simulink model "HyQ2Max_Leg_2Dof_ForAc1CylMot"  (Simulink 7.0)
settings: Solver=ode15s  StartTime=0.0  StopTime=10.0  MaxStep=1e-2  RelTol=1e-3
values from neighbouring files (symbols this model uses):
  L_LegInertiab_CAD = [ ... (first row only)    [HyQ2Max_CAD_For_SimMechanics_LF_RF.m]
  L_LegMb = 1.406    [HyQ2Max_CAD_For_SimMechanics_LF_RF.m]
  U_LegInertia_CAD = [0.010196 0.002320 0.000141 ... (first row only)    [HyQ2Max_CAD_For_SimMechanics_LF_RF.m]
  U_LegM = 4.95    [HyQ2Max_CAD_For_SimMechanics_LF_RF.m]
undefined symbols (not defined in the file or in its folder): sigbuilder_block
libraries: mblibv1 x24, fl_lib x15, nesl_utility x6, simulink x2
settings Model: Creator=Gustavo  LastModifiedBy=Gustavo
settings SolverCC: SolverResetMethod=Robust
settings DebuggingCC: SaveWithParameterizedLinksMsg=none  SignalResolutionControl=TryResolveAllWithWarning  MultiTaskDSMMsg=warning  MultiTaskCondExecSysMsg=none
settings RTWCC: IncludeERTFirstTime=on
settings GRTTargetCC: TargetFcnLib=ansi_tfl_tmw.mat
settings SimMechanicsCC: VisOnUpdateDiagram=on  VisDuringSimulation=on

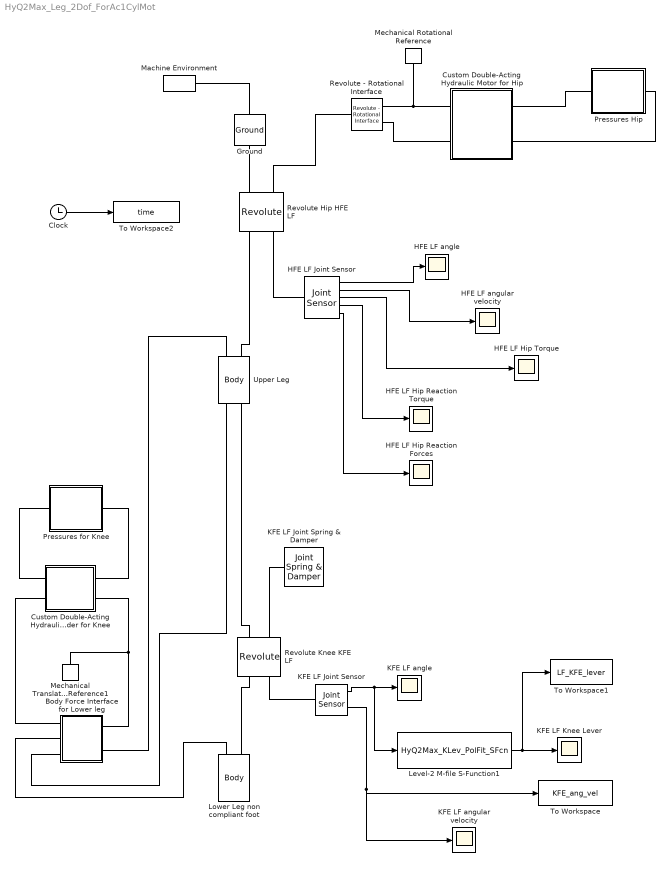
== system HyQ2Max_Leg_2Dof_ForAc1CylMot ==
  Body Force Interface for Lower leg : Subsystem
  Clock : Clock
      settings: Decimation=10
  Custom Double-Acting Hydraulic Cylinder for Knee : Subsystem  Orientation=left  mask(Hydraulic Double-Acting Cylinder, Custom Model){area_A=3.14e-004, area_B=2.00e-004, stroke=0.06834, init_pos=-1.4570e-4, stiffness=1e7, damping=1e5}
      mask prompts: area_A "Area A (m^2)"; area_B "Area B (m^2)"; stroke "Stroke (m)"; init_pos "Initial position (m)"; stiffness "Contact stiffness (N/m)"; damping "Contact damping (N*s/m)"
      mask help: The model is built entirely of Foundation Library blocks and accounts for hard stops and fluid consumption due to piston motion.
      mask Display:
      | plot([127.790967235342;156.136468285695;156.136468285695;127.790967235342;127.790967235342], [113.618216710165;113.618216710165;56.927214609459;56.927214609459;113.618216710165])
      | plot([227.000220911577;227.000220911577;56.927214609459;56.927214609459;227.000220911577;227.000220911577], [99.4454661849886;113.618216710165;113.618216710165;56.927214609459;56.927214609459;71.0999651346356])
      | plot([156.136468285695;297.86397353746;297.86397353746;156.136468285695;156.136468285695], [99.4454661849886;99.4454661849886;71.0999651346356;71.0999651346356;99.4454661849886])
      | plot([56.927214609459;28.581713559106;56.927214609459], [113.618216710165;85.2727156598121;56.927214609459])
      | plot([28.581713559106;0.236212508752942], [85.2727156598121;85.2727156598121])
      | plot([297.86397353746;326.209474587813], [85.2727156598121;85.2727156598121])
      | plot([0.236212508752942;71.0999651346356;71.0999651346356], [28.581713559106;28.581713559106;56.927214609459])
      | plot([212.827470386401;212.827470386401;323.374924482778], [56.927214609459;28.581713559106;28.581713559106])
      | patch([0;326.445687096566;326.445687096566;0;0;0.472425017505884;0.472425017505884;325.97326207906;325.97326207906;0.472425017505884;0], [113.854429218918;113.854429218918;0;0;113.854429218918;113.382004201412;0.472425017505884;0.472425017505884;113.382004201412;113.382004201412;113.854429218918], [1;1;1])
      | ;
  Custom Double-Acting Hydraulic Motor for Hip : Subsystem  Orientation=left  mask(Hydraulic Double-Acting Cylinder, Custom Model){Displacement=1.432e-5, stroke=270/180*pi, init_pos=135/180*pi, stiffness=1e7, damping=1e5, Damping_Coef=1.5}
      mask prompts: Displacement "Displacement (m^3/rad)"; stroke "Stroke (rad)"; init_pos "Initial position (rad)"; stiffness "Contact stiffness (Nm/rad)"; damping "Contact damping (Nm*s/rad)"; Damping_Coef "Damping Coef (Nm*s/rad)"
      mask help: The model is built entirely of Foundation Library blocks and accounts for hard stops and fluid consumption due to piston motion.
      mask Display:
      | plot([73.6992110911092;78.3372264117062;83.4855098283815;89.0944805574945;95.1101211447486;101.474497682805;108.12631774648;115.001520672305;122.033894497737;129.15571361855;136.298391023429;143.39313882438;150.371630721695;157.166660023573;163.712786883295;169.946968520725;175.809166358744;181.242924227569;186.195912068529;190.620429901137;194.473867199977;197.719113257359;200.324914579718;202.266175875843;203.524201738252;204.086876690183;203.948781864259;203.111247189144;201.582338581603;199.376780267312;196.51581297852;193.02698939418;188.943908792596;184.305893471999;179.157610055324;173.548639326211;167.532998738957;161.1686222009;154.516802137226;147.6415992114;140.609225385968;133.487406265155;126.344728860276;119.249981059326;112.27148916201;105.476459860132;98.9303330004107;92.6961513629807;86.8339535249614;81.4001956561362;76.4472078151762;72.0226899825683;70.8644989508936], [212.831540230622;218.265298099447;223.218285940407;227.642803773015;231.496241071855;234.741487129237;237.347288451596;239.288549747721;240.54657561013;241.109250562061;240.971155736137;240.133621061022;238.604712453481;236.39915413919;233.538186850398;230.049363266058;225.966282664474;221.328267343877;216.179983927202;210.571013198089;204.555372610835;198.190996072778;191.539176009104;184.663973083278;177.631599257846;170.509780137033;163.367102732154;156.272354931204;149.293863033888;142.49883373201;135.952706872289;129.718525234859;123.856327396839;118.422569528014;113.469581687054;109.045063854446;105.191626555606;101.946380498224;99.3405791758655;97.3993178797401;96.1412920173311;95.5786170654003;95.7167118913243;96.5542465664391;98.0831551739803;100.288713488271;103.149680777063;106.638504361403;110.721584962987;115.359600283584;120.50788370026;126.116854429373;127.792411177503])
      | plot([0;133.223854936659;133.223854936659], [255.34572196193;255.34572196193;241.172971436754])
      | plot([73.6983027309179;133.223854936659;70.8637526258826], [212.827470386401;170.309218810871;127.790967235342])
      | patch([110.547454096377;153.065705671906;133.223854936659;110.547454096377], [238.338421331719;238.338421331719;209.992920281366;238.338421331719], [0;0;0])
      | plot([110.547454096377;153.065705671906;133.223854936659;110.547454096377], [238.338421331719;238.338421331719;209.992920281366;238.338421331719])
      | patch([110.547454096377;153.065705671906;133.223854936659;110.547454096377], [99.4454661849887;99.4454661849887;127.790967235342;99.4454661849887], [0;0;0])
      | plot([110.547454096377;153.065705671906;133.223854936659;110.547454096377], [99.4454661849887;99.4454661849887;127.790967235342;99.4454661849887])
      | plot([204.087607562542;240.936758928001;240.936758928001;204.087607562542;204.087607562542], [178.812869125977;178.812869125977;161.805568495765;161.805568495765;178.812869125977])
      | plot([5.66910021007061;133.223854936659;133.223854936659], [85.2727156598121;85.2727156598121;96.6109160799534])
      | plot([240.936758928001;283.455010503531], [170.309218810871;170.309218810871])
      | patch([2.59833759628236;286.525773117319;286.525773117319;2.59833759628236;2.59833759628236;3.07076261378825;3.07076261378825;286.053348099813;286.053348099813;3.07076261378825;2.59833759628236], [340.618437621743;340.618437621743;0;5.6843418860808e-14;340.618437621743;340.146012604237;0.472425017505941;0.472425017505884;340.146012604237;340.146012604237;340.618437621743], [1;1;1])
      | ;color('red');
  Ground : mblibv1/Bodies/Ground  Orientation=down  DialogController=MECH.DynMechDlgSource  SystemSampleTime=-1  LeftPortType=env  RightPortType=workingframe  PhysicalDomain=Mechanical  DialogClass=GroundBlock  CoordPosition=[0 0 0]  CoordPositionUnits=m  StateVectorMgrId=-1  MachineId=[0 0]  ShowEnvPort=on
  HFE LF Joint Sensor : mblibv1/Sensors &  Actuators/Joint Sensor  DialogController=MECH.DynMechDlgSource  SystemSampleTime=-1  PhysicalDomain=Mechanical  PortType=blob  Muxed=off  Pose=off  Angle=on  AngleUnits=rad  ArcVelocity=on  ArcVelocityUnits=rad/s  ArcAcceleration=off  ArcAccelerationUnits=rad/s^2  CoordPosition=on  CoordPositionUnits=m  Velocity=off  VelocityUnits=m/s  Acceleration=off  AccelerationUnits=m/s^2  Quaternion=on  QuaternionDT=off  QuaternionDDT=off  QuaternionUnits=off  OutputVector=[ 1 ]  ActiveIO=on  Width=9  DialogClass=MechanicalSensorBlock  Primitive=R1  Force=off  ForceUnits=N  Torque=on  TorqueUnits=N*m  ReferenceFrame=Absolute (INERTIAL)  ReactionSensedSide=Base  ReactionReferenceFrame=Absolute (World)  ReactionForce=on  ReactionForceUnits=N  ReactionMoment=on  ReactionMomentUnits=N*m
  HFE LF angular velocity : Scope
      settings: YMin=-2.5  YMax=0.25  SaveName=ScopeData10
  HFE LF Hip Reaction Forces : Scope
      settings: TimeRange=10  YMin=-40  YMax=40  SaveName=ScopeData6
  HFE LF Hip Reaction Torque : Scope
      settings: TimeRange=10  YMin=-0.4  YMax=0.3  SaveName=ScopeData7
  HFE LF Hip Torque : Scope
      settings: TimeRange=10  YMin=-7.5  YMax=7.5  SaveName=ScopeData4
  HFE LF angle : Scope
      settings: YMin=-2.5  YMax=0.25
  KFE LF Joint Sensor : mblibv1/Sensors &  Actuators/Joint Sensor  DialogController=MECH.DynMechDlgSource  SystemSampleTime=-1  PhysicalDomain=Mechanical  PortType=blob  Muxed=off  Pose=off  Angle=on  AngleUnits=rad  ArcVelocity=on  ArcVelocityUnits=rad/s  ArcAcceleration=off  ArcAccelerationUnits=rad/s^2  CoordPosition=on  CoordPositionUnits=m  Velocity=off  VelocityUnits=m/s  Acceleration=off  AccelerationUnits=m/s^2  Quaternion=on  QuaternionDT=off  QuaternionDDT=off  QuaternionUnits=off  OutputVector=[ 1 ]  ActiveIO=on  Width=2  DialogClass=MechanicalSensorBlock  Primitive=R1  Force=off  ForceUnits=N  Torque=off  TorqueUnits=N*m  ReferenceFrame=Absolute (INERTIAL)  ReactionSensedSide=Base  ReactionReferenceFrame=Absolute (World)  ReactionForce=off  ReactionForceUnits=N  ReactionMoment=off  ReactionMomentUnits=N*m
  KFE LF Joint Spring & Damper : mblibv1/Force  Elements/Joint Spring & Damper  DialogController=MECH.DynMechDlgSource  SystemSampleTime=-1  DialogClass=JointSpringDamper  JFEParameters=P1$false$0$0$0$m$m/s$N$deg$deg/s$N*m#P2$false$0$0$0$m$m/s$N$deg$deg/s$N*m#P3$false$0$0$0$m$m/s$N$deg$deg/s$N*m#R1$true$0$0.5$0$m$m/s$N$rad$rad/s$N*m#R2$false$0$0$0$m$m/s$N$deg$deg/s$N*m#R3$false$0$0$0$m$m/s$N$deg$deg/s$N*m#S$false$0$0$0$m$m/s$N$deg$deg/s$N*m
  KFE LF Knee Lever : Scope
      settings: TimeRange=10  YMin=0.005  YMax=0.04  SaveName=ScopeData9
  KFE LF angle : Scope
      settings: YMin=-3.5  YMax=3.5  SaveName=ScopeData8
  KFE LF angular velocity : Scope
      settings: YMin=-3.5  YMax=3.5
  Level-2 M-file S-Function1 : M-S-Function  FunctionName=HyQ2Max_KLev_PolFit_SFcn
  Lower Leg non compliant foot : mblibv1/Bodies/Body  Orientation=down  DialogController=MECH.DynMechDlgSource  PhysicalDomain=mechanical  SubClassName=Unknown  LeftPortType=workingframe  RightPortType=workingframe  LConnTagsString=CS3|CS1  RConnTagsString=CS2  DialogClass=MechanicalBodyBlock  Mass=L_LegMb  MassUnits=kg  InertiaUnits=kg*m^2  Inertia=L_LegInertiab_CAD  Shape=Cylinder  ShapeDims=[1 1]  ShapeUnits=m  ShapeUse=false  Density=1  DensityUnits=kg/m^3  DensityUse=false  CG=Left$CG$L_LegCogb_CAD$CS1$CS1$m$[-90 180 0]$Euler Z-X-Z$deg$World$false  WorkingFrames="Left$CS3$[0.0262 0.0216 0]$CS1$CS1$m$[-90 180 0]$Euler Z-X-Z$deg$World$true#Left$CS1$[0 0  0]$Adjoining$Adjoining$m$[-90 180 0]$Euler Z-X-Z$deg$World$true#Right$CS2$[0.38009 0 0]$CS1$CS1$m$[-90 180 0]$Euler Z-X-Z$deg$World$true"  CGPos=L_LegCogb_CAD  CGRot=[-90 180 0]  CS0Pos=[]  CS0Rot=[]  CS1Pos="[0 0  0]"  CS1Rot=[-90 180 0]  CS2Pos=[0.38009 0 0]  CS2Rot=[-90 180 0]  CS3Pos=[0.0262 0.0216 0]  CS3Rot=[-90 180 0]  CS4Pos=[]  CS4Rot=[]  CS5Pos=[]  CS5Rot=[]  CS6Pos=[]  CS6Rot=[]  CS7Pos=[]  CS7Rot=[]  CS8Pos=[]  CS8Rot=[]  CS9Pos=[]  CS9Rot=[]  CS10Pos=[]  CS10Rot=[]  CS11Pos=[]  CS11Rot=[]  CS12Pos=[]  CS12Rot=[]  CS13Pos=[]  CS13Rot=[]  CS14Pos=[]  CS14Rot=[]  CS15Pos=[]  CS15Rot=[]  CS16Pos=[]  CS16Rot=[]  CS17Pos=[]  CS17Rot=[]  CS18Pos=[]  CS18Rot=[]  CS19Pos=[]  CS19Rot=[]  CS20Pos=[]  CS20Rot=[]
  Machine Environment : mblibv1/Bodies/Machine Environment  Tag=Factory ground  DialogController=MECH.DialogSource  SystemSampleTime=-1  PortType=env  PhysicalDomain=Mechanical  DialogTemplateClass=MECH.MachineEnvironment  SyncWhenCopied=off  Gravity=[0 -9.81 0]  GravityUnits=m/s^2  GravityAsSignal=off  Dimensionality=Auto-detect  AnalysisType=Forward dynamics  LinearAssemblyTolerance=1e-3  LinearAssemblyToleranceUnits=m  AngularAssemblyTolerance=1e-3  AngularAssemblyToleranceUnits=rad  ConstraintSolverType=Stabilizing  ConstraintRelTolerance=1e-4  ConstraintAbsTolerance=1e-4  UseRobustSingularityHandling=off  RedundancyAnalysisToleranceType=Automatically select tolerance  RedundancyAnalysisTolerance=1e-14  StatePerturbationType=Fixed  PerturbationSize=1e-5  VisualizeMachine=on
  Mechanical Rotational Reference : fl_lib/Mechanical/Rotational Elements/Mechanical Rotational Reference  Orientation=up  DialogController=NetworkEngine.DynNeDlgSource  SystemSampleTime=-1  LocalVarLogging=[]
  Mechanical Translational Reference1 : fl_lib/Mechanical/Translational Elements/Mechanical Translational Reference  Orientation=down  DialogController=NetworkEngine.DynNeDlgSource  SystemSampleTime=-1  LocalVarLogging=[]
  Pressures for Knee : Subsystem
  Pressures Hip : Subsystem  Orientation=left
  Revolute Hip HFE LF : mblibv1/Joints/Revolute  Orientation=down  DialogController=MECH.DynMechDlgSource  PhysicalDomain=mechanical  SubClassName=Unknown  LeftPortType=blob  RightPortType=blob  LConnTagsString=__newl0|SA1  RConnTagsString=__newr0|SA1  NumSAPorts=2  CutJoint=off  MarkAsCut=off  Primitives=revolute  PrimitiveProps=R1$World$[0 0 -1]$revolute  DialogClass=JointBlock  R1Axis=[0 0 -1]
  Revolute Knee KFE LF : mblibv1/Joints/Revolute  Orientation=down  DialogController=MECH.DynMechDlgSource  PhysicalDomain=mechanical  SubClassName=Unknown  LeftPortType=blob  RightPortType=blob  LConnTagsString=__newl0|SA1  RConnTagsString=__newr0|SA1  NumSAPorts=2  CutJoint=off  MarkAsCut=off  Primitives=revolute  PrimitiveProps=R1$World$[0 0 -1]$revolute  DialogClass=JointBlock  R1Axis=[0 0 -1]
  Revolute - Rotational Interface : mblibv1/Interface  Elements/Revolute - Rotational Interface  Orientation=left  DialogController=MECH.DynMechDlgSource  SystemSampleTime=-1  DialogClass=RevoluteRotationalInterface  Primitive=R1
  To Workspace : ToWorkspace  VariableName=KFE_ang_vel  SampleTime=-1  SaveFormat=Array
  To Workspace1 : ToWorkspace  VariableName=LF_KFE_lever  SampleTime=-1  SaveFormat=Array
  To Workspace2 : ToWorkspace  VariableName=time  SampleTime=-1  SaveFormat=Array
  Upper Leg : mblibv1/Bodies/Body  Orientation=down  DialogController=MECH.DynMechDlgSource  PhysicalDomain=mechanical  SubClassName=Unknown  LeftPortType=workingframe  RightPortType=workingframe  LConnTagsString=CS4|CS1  RConnTagsString=CS3|CS2  DialogClass=MechanicalBodyBlock  Mass=U_LegM  MassUnits=kg  InertiaUnits=kg*m^2  Inertia=U_LegInertia_CAD  Shape=Cylinder  ShapeDims=[1 1]  ShapeUnits=m  ShapeUse=false  Density=1  DensityUnits=kg/m^3  DensityUse=false  CG=Left$CG$U_LegCog_CAD$CS1$CS1$m$[-90 180 0]$Euler Z-X-Z$deg$WORLD$false  WorkingFrames="Left$CS4$[-.041 -.005 0]$CS1$CS1$m$[-90 180 0]$Euler Z-X-Z$deg$WORLD$true#Right$CS3$[.32  .023 0]$CS1$CS1$m$[-90 180 0]$Euler Z-X-Z$deg$WORLD$true#Left$CS1$[0 0 0]$World$World$m$[-90 180 0]$Euler Z-X-Z$deg$World$true#Right$CS2$[.36 0 0]$CS1$CS1$m$[-90 180 0]$Euler Z-X-Z$deg$World$true"  CGPos=U_LegCog_CAD  CGRot=[-90 180 0]  CS0Pos=[]  CS0Rot=[]  CS1Pos=[0 0 0]  CS1Rot=[-90 180 0]  CS2Pos=[.36 0 0]  CS2Rot=[-90 180 0]  CS3Pos="[.32  .023 0]"  CS3Rot=[-90 180 0]  CS4Pos=[-.041 -.005 0]  CS4Rot=[-90 180 0]  CS5Pos=[]  CS5Rot=[]  CS6Pos=[]  CS6Rot=[]  CS7Pos=[]  CS7Rot=[]  CS8Pos=[]  CS8Rot=[]  CS9Pos=[]  CS9Rot=[]  CS10Pos=[]  CS10Rot=[]  CS11Pos=[]  CS11Rot=[]  CS12Pos=[]  CS12Rot=[]  CS13Pos=[]  CS13Rot=[]  CS14Pos=[]  CS14Rot=[]  CS15Pos=[]  CS15Rot=[]  CS16Pos=[]  CS16Rot=[]  CS17Pos=[]  CS17Rot=[]  CS18Pos=[]  CS18Rot=[]  CS19Pos=[]  CS19Rot=[]  CS20Pos=[]  CS20Rot=[]
  wires:
  HFE LF Joint Sensor/1 -> HFE LF angle/1
  KFE LF Joint Sensor/1 -> KFE LF angle/1, Level-2 M-file S-Function1/1
  Level-2 M-file S-Function1/1 -> KFE LF Knee Lever/1, To Workspace1/1
  HFE LF Joint Sensor/5 -> HFE LF Hip Reaction Forces/1
  HFE LF Joint Sensor/4 -> HFE LF Hip Reaction Torque/1
  HFE LF Joint Sensor/3 -> HFE LF Hip Torque/1
  HFE LF Joint Sensor/2 -> HFE LF angular velocity/1
  KFE LF Joint Sensor/2 -> KFE LF angular velocity/1, To Workspace/1
  Clock/1 -> To Workspace2/1
  connections:
  HFE LF Joint Sensor/LConn1 -- Revolute Hip HFE LF/RConn2
  Machine Environment/RConn1 -- Ground/LConn1
  Ground/RConn1 -- Revolute Hip HFE LF/LConn1
  Revolute Hip HFE LF/RConn1 -- Upper Leg/LConn2
  Upper Leg/RConn2 -- Revolute Knee KFE LF/LConn1
  KFE LF Joint Sensor/LConn1 -- Revolute Knee KFE LF/RConn2
  Lower Leg non compliant foot/LConn2 -- Revolute Knee KFE LF/RConn1
  Lower Leg non compliant foot/LConn1 -- Body Force Interface for Lower leg/LConn2
  Revolute Knee KFE LF/LConn2 -- KFE LF Joint Spring & Damper/LConn1
  Body Force Interface for Lower leg/RConn2 -- Upper Leg/LConn1
  Upper Leg/RConn1 -- Body Force Interface for Lower leg/LConn3
  Pressures for Knee/LConn1 -- Custom Double-Acting Hydraulic Cylinder for Knee/RConn1
  Pressures for Knee/RConn1 -- Custom Double-Acting Hydraulic Cylinder for Knee/LConn1
  Body Force Interface for Lower leg/RConn1 -- Custom Double-Acting Hydraulic Cylinder for Knee/LConn2 -- Mechanical Translational Reference1/LConn1
  Custom Double-Acting Hydraulic Cylinder for Knee/RConn2 -- Body Force Interface for Lower leg/LConn1
  Custom Double-Acting Hydraulic Motor for Hip/LConn2 -- Pressures Hip/LConn1
  Revolute - Rotational Interface/LConn2 -- Custom Double-Acting Hydraulic Motor for Hip/RConn2
  Revolute - Rotational Interface/LConn1 -- Custom Double-Acting Hydraulic Motor for Hip/RConn1 -- Mechanical Rotational Reference/LConn1
  Pressures Hip/RConn1 -- Custom Double-Acting Hydraulic Motor for Hip/LConn1
  Revolute - Rotational Interface/RConn1 -- Revolute Hip HFE LF/LConn2

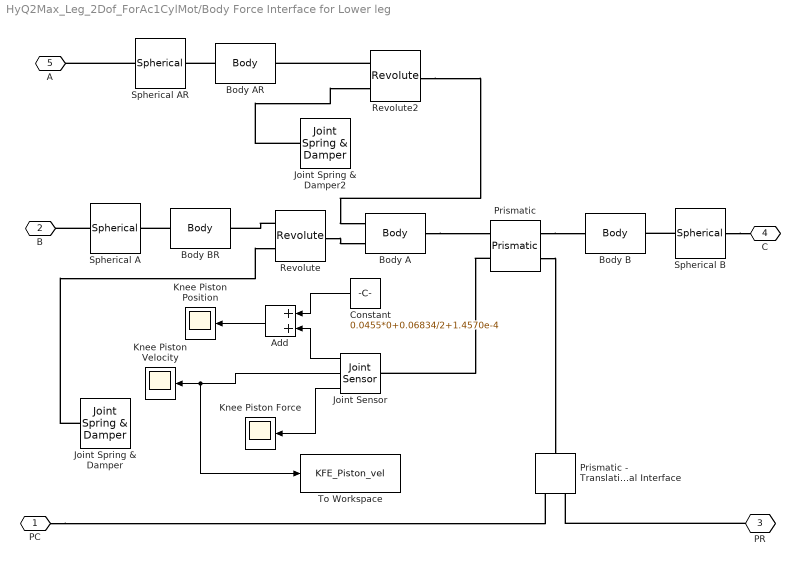
== system HyQ2Max_Leg_2Dof_ForAc1CylMot/Body Force Interface for Lower leg ==
  Add : Sum  Orientation=left  OutDataType=sfix(16)  OutScaling=2^-10
  Body A : mblibv1/Bodies/Body  DialogController=MECH.DynMechDlgSource  PhysicalDomain=mechanical  SubClassName=Unknown  LeftPortType=workingframe  RightPortType=workingframe  LConnTagsString=CS3|CS1  RConnTagsString=CS2  DialogClass=MechanicalBodyBlock  Mass=0.09  MassUnits=kg  InertiaUnits=kg*m^2  Inertia=eye(3)*1e-4  Shape=Cylinder  ShapeDims=[1 1]  ShapeUnits=m  ShapeUse=false  Density=1  DensityUnits=kg/m^3  DensityUse=false  CG=Left$CG$[-.3935857/2 0 0]$CS1$CS1$m$[0 0 0]$Euler X-Y-Z$deg$CS1$false  WorkingFrames=Left$CS3$[0 0 0]$Adjoining$Adjoining$m$[0 0 0]$Euler X-Y-Z$deg$Adjoining$true#Left$CS1$[0 0 0]$Adjoining$Adjoining$m$[0 0 -55.1441]$Euler X-Y-Z$deg$Adjoining$true#Right$CS2$[-.3935857 0 0]$CS1$CS1$m$[0 0 0]$Euler X-Y-Z$deg$CS1$true  CGPos=[-.3935857/2 0 0]  CGRot=[0 0 0]  CS0Pos=[]  CS0Rot=[]  CS1Pos=[0 0 0]  CS1Rot=[0 0 -55.1441]  CS2Pos=[-.3935857 0 0]  CS2Rot=[0 0 0]  CS3Pos=[0 0 0]  CS3Rot=[0 0 0]  CS4Pos=[]  CS4Rot=[]  CS5Pos=[]  CS5Rot=[]  CS6Pos=[]  CS6Rot=[]  CS7Pos=[]  CS7Rot=[]  CS8Pos=[]  CS8Rot=[]  CS9Pos=[]  CS9Rot=[]  CS10Pos=[]  CS10Rot=[]  CS11Pos=[]  CS11Rot=[]  CS12Pos=[]  CS12Rot=[]  CS13Pos=[]  CS13Rot=[]  CS14Pos=[]  CS14Rot=[]  CS15Pos=[]  CS15Rot=[]  CS16Pos=[]  CS16Rot=[]  CS17Pos=[]  CS17Rot=[]  CS18Pos=[]  CS18Rot=[]  CS19Pos=[]  CS19Rot=[]  CS20Pos=[]  CS20Rot=[]
  Body AR : mblibv1/Bodies/Body  DialogController=MECH.DynMechDlgSource  PhysicalDomain=mechanical  SubClassName=Unknown  LeftPortType=workingframe  RightPortType=workingframe  LConnTagsString=CS1  RConnTagsString=CS2  DialogClass=MechanicalBodyBlock  Mass=0.01  MassUnits=kg  InertiaUnits=kg*m^2  Inertia=eye(3)*1e-3  Shape=Cylinder  ShapeDims=[1 1]  ShapeUnits=m  ShapeUse=false  Density=1  DensityUnits=kg/m^3  DensityUse=false  CG=Left$CG$[.056/2 0 0]$CS1$CS1$m$[0 0 0]$Euler X-Y-Z$deg$CS1$false  WorkingFrames=Left$CS1$[0 0 0]$Adjoining$Adjoining$m$[0 0 -52.3270]$Euler X-Y-Z$deg$Adjoining$true#Right$CS2$[.056 0 0]$CS1$CS1$m$[0 0 0]$Euler X-Y-Z$deg$CS1$true  CGPos=[.056/2 0 0]  CGRot=[0 0 0]  CS0Pos=[]  CS0Rot=[]  CS1Pos=[0 0 0]  CS1Rot=[0 0 -52.3270]  CS2Pos=[.056 0 0]  CS2Rot=[0 0 0]  CS3Pos=[]  CS3Rot=[]  CS4Pos=[]  CS4Rot=[]  CS5Pos=[]  CS5Rot=[]  CS6Pos=[]  CS6Rot=[]  CS7Pos=[]  CS7Rot=[]  CS8Pos=[]  CS8Rot=[]  CS9Pos=[]  CS9Rot=[]  CS10Pos=[]  CS10Rot=[]  CS11Pos=[]  CS11Rot=[]  CS12Pos=[]  CS12Rot=[]  CS13Pos=[]  CS13Rot=[]  CS14Pos=[]  CS14Rot=[]  CS15Pos=[]  CS15Rot=[]  CS16Pos=[]  CS16Rot=[]  CS17Pos=[]  CS17Rot=[]  CS18Pos=[]  CS18Rot=[]  CS19Pos=[]  CS19Rot=[]  CS20Pos=[]  CS20Rot=[]
  Body B : mblibv1/Bodies/Body  DialogController=MECH.DynMechDlgSource  PhysicalDomain=mechanical  SubClassName=Unknown  LeftPortType=workingframe  RightPortType=workingframe  LConnTagsString=CS1  RConnTagsString=CS2  DialogClass=MechanicalBodyBlock  Mass=0.09  MassUnits=kg  InertiaUnits=kg*m^2  Inertia=eye(3)*1e-4  Shape=Cylinder  ShapeDims=[1 1]  ShapeUnits=m  ShapeUse=false  Density=1  DensityUnits=kg/m^3  DensityUse=false  CG=Left$CG$[-.3935857/2 0 0]$CS1$CS1$m$[0 0 0]$Euler X-Y-Z$deg$CS1$false  WorkingFrames=Left$CS1$[.3935857 0 0]$Adjoining$Adjoining$m$[0 0 0]$Euler X-Y-Z$deg$Adjoining$true#Right$CS2$[-.3935857 0 0]$CS1$CS1$m$[0 0 0]$Euler X-Y-Z$deg$CS1$true  CGPos=[-.3935857/2 0 0]  CGRot=[0 0 0]  CS0Pos=[]  CS0Rot=[]  CS1Pos=[.3935857 0 0]  CS1Rot=[0 0 0]  CS2Pos=[-.3935857 0 0]  CS2Rot=[0 0 0]  CS3Pos=[]  CS3Rot=[]  CS4Pos=[]  CS4Rot=[]  CS5Pos=[]  CS5Rot=[]  CS6Pos=[]  CS6Rot=[]  CS7Pos=[]  CS7Rot=[]  CS8Pos=[]  CS8Rot=[]  CS9Pos=[]  CS9Rot=[]  CS10Pos=[]  CS10Rot=[]  CS11Pos=[]  CS11Rot=[]  CS12Pos=[]  CS12Rot=[]  CS13Pos=[]  CS13Rot=[]  CS14Pos=[]  CS14Rot=[]  CS15Pos=[]  CS15Rot=[]  CS16Pos=[]  CS16Rot=[]  CS17Pos=[]  CS17Rot=[]  CS18Pos=[]  CS18Rot=[]  CS19Pos=[]  CS19Rot=[]  CS20Pos=[]  CS20Rot=[]
  Body BR : mblibv1/Bodies/Body  DialogController=MECH.DynMechDlgSource  PhysicalDomain=mechanical  SubClassName=Unknown  LeftPortType=workingframe  RightPortType=workingframe  LConnTagsString=CS1  RConnTagsString=CS2  DialogClass=MechanicalBodyBlock  Mass=0.01  MassUnits=kg  InertiaUnits=kg*m^2  Inertia=eye(3)*1e-3  Shape=Cylinder  ShapeDims=[1 1]  ShapeUnits=m  ShapeUse=false  Density=1  DensityUnits=kg/m^3  DensityUse=false  CG=Left$CG$[-.056/2 0 0]$CS1$CS1$m$[0 0 0]$Euler X-Y-Z$deg$CS1$false  WorkingFrames=Left$CS1$[0 0 0]$Adjoining$Adjoining$m$[0 0 52.5477]$Euler X-Y-Z$deg$Adjoining$true#Right$CS2$[-.056 0 0]$CS1$CS1$m$[0 0 0]$Euler X-Y-Z$deg$CS1$true  CGPos=[-.056/2 0 0]  CGRot=[0 0 0]  CS0Pos=[]  CS0Rot=[]  CS1Pos=[0 0 0]  CS1Rot=[0 0 52.5477]  CS2Pos=[-.056 0 0]  CS2Rot=[0 0 0]  CS3Pos=[]  CS3Rot=[]  CS4Pos=[]  CS4Rot=[]  CS5Pos=[]  CS5Rot=[]  CS6Pos=[]  CS6Rot=[]  CS7Pos=[]  CS7Rot=[]  CS8Pos=[]  CS8Rot=[]  CS9Pos=[]  CS9Rot=[]  CS10Pos=[]  CS10Rot=[]  CS11Pos=[]  CS11Rot=[]  CS12Pos=[]  CS12Rot=[]  CS13Pos=[]  CS13Rot=[]  CS14Pos=[]  CS14Rot=[]  CS15Pos=[]  CS15Rot=[]  CS16Pos=[]  CS16Rot=[]  CS17Pos=[]  CS17Rot=[]  CS18Pos=[]  CS18Rot=[]  CS19Pos=[]  CS19Rot=[]  CS20Pos=[]  CS20Rot=[]
  Constant : Constant  Orientation=left  Value=0.0455*0+0.06834/2+1.4570e-4  OutDataType=sfix(16)  OutScaling=2^0
  Joint Spring & Damper : mblibv1/Force  Elements/Joint Spring & Damper  DialogController=MECH.DynMechDlgSource  SystemSampleTime=-1  DialogClass=JointSpringDamper  JFEParameters=P1$false$0$0$0$m$m/s$N$deg$deg/s$N*m#P2$false$0$0$0$m$m/s$N$deg$deg/s$N*m#P3$false$0$0$0$m$m/s$N$deg$deg/s$N*m#R1$false$0$0.5$0$m$m/s$N$rad$rad/s$N*m#R2$false$0$0$0$m$m/s$N$deg$deg/s$N*m#R3$false$0$0$0$m$m/s$N$deg$deg/s$N*m#S$false$0$0$0$m$m/s$N$deg$deg/s$N*m
  Joint Spring & Damper2 : mblibv1/Force  Elements/Joint Spring & Damper  DialogController=MECH.DynMechDlgSource  SystemSampleTime=-1  DialogClass=JointSpringDamper  JFEParameters=P1$false$0$0$0$m$m/s$N$deg$deg/s$N*m#P2$false$0$0$0$m$m/s$N$deg$deg/s$N*m#P3$false$0$0$0$m$m/s$N$deg$deg/s$N*m#R1$false$0$0.5$0$m$m/s$N$rad$rad/s$N*m#R2$false$0$0$0$m$m/s$N$deg$deg/s$N*m#R3$false$0$0$0$m$m/s$N$deg$deg/s$N*m#S$false$0$0$0$m$m/s$N$deg$deg/s$N*m
  Joint Sensor : mblibv1/Sensors &  Actuators/Joint Sensor  Orientation=left  DialogController=MECH.DynMechDlgSource  SystemSampleTime=-1  PhysicalDomain=Mechanical  PortType=blob  Muxed=off  Pose=off  Angle=on  AngleUnits=deg  ArcVelocity=off  ArcVelocityUnits=deg/s  ArcAcceleration=off  ArcAccelerationUnits=deg/s^2  CoordPosition=on  CoordPositionUnits=m  Velocity=on  VelocityUnits=m/s  Acceleration=off  AccelerationUnits=m/s^2  Quaternion=on  QuaternionDT=off  QuaternionDDT=off  QuaternionUnits=off  OutputVector=[1]  ActiveIO=on  Width=3  DialogClass=MechanicalSensorBlock  Primitive=P1  Force=on  ForceUnits=N  Torque=off  TorqueUnits=N*m  ReferenceFrame=Absolute (World)  ReactionSensedSide=Base  ReactionReferenceFrame=Absolute (World)  ReactionForce=off  ReactionForceUnits=N  ReactionMoment=off  ReactionMomentUnits=N*m
  Knee Piston Force : Scope
      settings: TimeRange=10  YMin=-100  YMax=100  SaveName=ScopeData2
  Knee Piston Position : Scope
      settings: YMin=-0.035  YMax=0.035  SaveName=ScopeData3
  Knee Piston Velocity : Scope
      settings: YMin=-0.035  YMax=0.035  SaveName=ScopeData5
  Prismatic : mblibv1/Joints/Prismatic  Orientation=left  DialogController=MECH.DynMechDlgSource  PhysicalDomain=mechanical  SubClassName=Unknown  LeftPortType=blob  RightPortType=blob  LConnTagsString=__newl0|SA1  RConnTagsString=__newr0|SA1  NumSAPorts=2  CutJoint=off  MarkAsCut=off  Primitives=prismatic  PrimitiveProps=P1$Base$[1 0 0]$prismatic  DialogClass=JointBlock  P1Axis=[1 0 0]
  Prismatic - Translational Interface : mblibv1/Interface  Elements/Prismatic - Translational Interface  Orientation=up  DialogController=MECH.DynMechDlgSource  SystemSampleTime=-1  DialogClass=PrismaticTranslationalInterface  Primitive=P1
  Revolute : mblibv1/Joints/Revolute  DialogController=MECH.DynMechDlgSource  PhysicalDomain=mechanical  SubClassName=Unknown  LeftPortType=blob  RightPortType=blob  LConnTagsString=__newl0|SA1  RConnTagsString=__newr0  NumSAPorts=1  CutJoint=off  MarkAsCut=off  Primitives=prismatic  PrimitiveProps=R1$Follower$[0 0 1]$revolute  DialogClass=JointBlock  R1Axis=[0 0 1]
  Revolute2 : mblibv1/Joints/Revolute  DialogController=MECH.DynMechDlgSource  PhysicalDomain=mechanical  SubClassName=Unknown  LeftPortType=blob  RightPortType=blob  LConnTagsString=__newl0|SA1  RConnTagsString=__newr0  NumSAPorts=1  CutJoint=off  MarkAsCut=off  Primitives=prismatic  PrimitiveProps=R1$Follower$[0 0 1]$revolute  DialogClass=JointBlock  R1Axis=[0 0 1]
  Spherical A : mblibv1/Joints/Spherical  DialogController=MECH.DynMechDlgSource  PhysicalDomain=mechanical  SubClassName=Unknown  LeftPortType=blob  RightPortType=blob  LConnTagsString=__newl0  RConnTagsString=__newr0  NumSAPorts=0  CutJoint=off  MarkAsCut=off  Primitives=spherical  PrimitiveProps=S$WORLD$[0 0 0]$spherical  DialogClass=JointBlock  SAxis=[0 0 0]
  Spherical AR : mblibv1/Joints/Spherical  DialogController=MECH.DynMechDlgSource  PhysicalDomain=mechanical  SubClassName=Unknown  LeftPortType=blob  RightPortType=blob  LConnTagsString=__newl0  RConnTagsString=__newr0  NumSAPorts=0  CutJoint=off  MarkAsCut=off  Primitives=spherical  PrimitiveProps=S$WORLD$[0 0 0]$spherical  DialogClass=JointBlock  SAxis=[0 0 0]
  Spherical B : mblibv1/Joints/Spherical  DialogController=MECH.DynMechDlgSource  PhysicalDomain=mechanical  SubClassName=Unknown  LeftPortType=blob  RightPortType=blob  LConnTagsString=__newl0  RConnTagsString=__newr0  NumSAPorts=0  CutJoint=off  MarkAsCut=off  Primitives=spherical  PrimitiveProps=S$WORLD$[0 0 0]$spherical  DialogClass=JointBlock  SAxis=[0 0 0]
  To Workspace : ToWorkspace  VariableName=KFE_Piston_vel  SampleTime=-1  SaveFormat=Array
  PC : PMIOPort  Port=1  Side=Left
  B : PMIOPort  Port=2  Side=Left
  PR : PMIOPort  Orientation=left  Port=3  Side=Right
  C : PMIOPort  Orientation=left  Port=4  Side=Right
  A : PMIOPort  Port=5  Side=Left
  wires:
  Constant/1 -> Add/1
  Add/1 -> Knee Piston Position/1
  Joint Sensor/1 -> Add/2
  Joint Sensor/3 -> Knee Piston Force/1
  Joint Sensor/2 -> Knee Piston Velocity/1, To Workspace/1
  connections:
  Body A/RConn1 -- Prismatic/RConn1
  Prismatic/LConn1 -- Body B/LConn1
  Spherical B/RConn1 -- C/RConn1
  Spherical B/LConn1 -- Body B/RConn1
  Prismatic/RConn2 -- Joint Sensor/LConn1
  Spherical A/LConn1 -- B/RConn1
  Body BR/LConn1 -- Spherical A/RConn1
  Revolute/RConn1 -- Body A/LConn2
  Revolute/LConn1 -- Body BR/RConn1
  Joint Spring & Damper/LConn1 -- Revolute/LConn2
  Spherical AR/LConn1 -- A/RConn1
  Body AR/LConn1 -- Spherical AR/RConn1
  Revolute2/RConn1 -- Body A/LConn1
  Revolute2/LConn1 -- Body AR/RConn1
  Joint Spring & Damper2/LConn1 -- Revolute2/LConn2
  PC/RConn1 -- Prismatic - Translational Interface/LConn1
  PR/RConn1 -- Prismatic - Translational Interface/LConn2
  Prismatic/LConn2 -- Prismatic - Translational Interface/RConn1

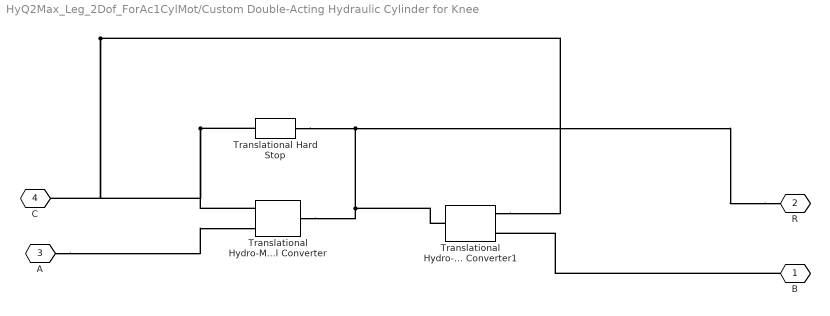
== system HyQ2Max_Leg_2Dof_ForAc1CylMot/Custom Double-Acting Hydraulic Cylinder for Knee ==
  Translational Hydro-Mechanical Converter : fl_lib/Hydraulic/Hydraulic Elements/Translational Hydro-Mechanical Converter  DialogController=NetworkEngine.DynNeDlgSource  SystemSampleTime=-1  area=area_A m^2  or=2  flow_rate_Log=off  pressure_Log=off  force_Log=off  power_Log=off  LocalVarNames=|flow_rate|pressure|force|power  LocalVarDescs=|Flow rate into the chamber (m^3/s)|Pressure at the inlet (Pa)|Output force (N)|Power (W)  LocalVarLogging=[0 0 0 0]
  Translational Hydro-Mechanical Converter1 : fl_lib/Hydraulic/Hydraulic Elements/Translational Hydro-Mechanical Converter  Orientation=left  DialogController=NetworkEngine.DynNeDlgSource  SystemSampleTime=-1  area=area_B m^2  or=1  flow_rate_Log=off  pressure_Log=off  force_Log=off  power_Log=off  LocalVarNames=|flow_rate|pressure|force|power  LocalVarDescs=|Flow rate into the chamber (m^3/s)|Pressure at the inlet (Pa)|Output force (N)|Power (W)  LocalVarLogging=[0 0 0 0]
  Translational Hard Stop : fl_lib/Mechanical/Translational Elements/Translational Hard Stop  Orientation=left  DialogController=NetworkEngine.DynNeDlgSource  SystemSampleTime=-1  upper_bnd=stroke - init_pos m  lower_bnd=-init_pos m  stiff_up=stiffness N/m  stiff_low=stiffness N/m  D_up=damping N/(m/s)  D_low=damping N/(m/s)  contact_force_Log=off  rel_displacement_Log=off  LocalVarNames=|contact_force|rel_displacement  LocalVarDescs=|Contact force (N)|Slider-case relative displacement (m)  LocalVarLogging=[0 0]
  B : PMIOPort  Tag=PMCPort  Orientation=left  Port=1  Side=Right
  R : PMIOPort  Tag=PMCPort  Orientation=left  Port=2  Side=Right
  A : PMIOPort  Tag=PMCPort  Port=3  Side=Left
  C : PMIOPort  Tag=PMCPort  Port=4  Side=Left
  connections:
  R/RConn1 -- Translational Hydro-Mechanical Converter1/RConn1 -- Translational Hydro-Mechanical Converter/RConn1 -- Translational Hard Stop/LConn1
  Translational Hydro-Mechanical Converter1/LConn1 -- Translational Hydro-Mechanical Converter/LConn1 -- Translational Hard Stop/RConn1 -- C/RConn1
  A/RConn1 -- Translational Hydro-Mechanical Converter/LConn2
  B/RConn1 -- Translational Hydro-Mechanical Converter1/LConn2

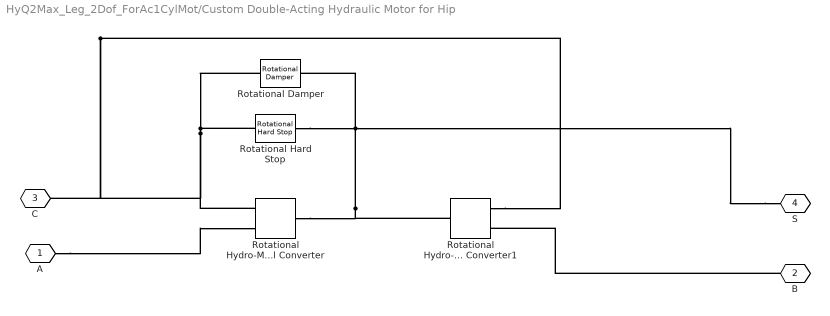
== system HyQ2Max_Leg_2Dof_ForAc1CylMot/Custom Double-Acting Hydraulic Motor for Hip ==
  Rotational Hydro-Mechanical Converter : fl_lib/Hydraulic/Hydraulic Elements/Rotational Hydro-Mechanical Converter  DialogController=NetworkEngine.DynNeDlgSource  SystemSampleTime=-1  D=Displacement m^3/rad  or=1  flow_rate_Log=off  pressure_Log=off  torque_Log=off  ang_velocity_Log=off  power_Log=off  LocalVarNames=|flow_rate|pressure|torque|ang_velocity|power  LocalVarDescs=|Flow rate into the chamber (m^3/s)|Pressure at the inlet (Pa)|Output torque (N*m)|Shaft angular velocity (rad/s)|Power (W)  LocalVarLogging=[0 0 0 0 0]
  Rotational Hydro-Mechanical Converter1 : fl_lib/Hydraulic/Hydraulic Elements/Rotational Hydro-Mechanical Converter  Orientation=left  DialogController=NetworkEngine.DynNeDlgSource  SystemSampleTime=-1  D=Displacement m^3/rad  or=2  flow_rate_Log=off  pressure_Log=off  torque_Log=off  ang_velocity_Log=off  power_Log=off  LocalVarNames=|flow_rate|pressure|torque|ang_velocity|power  LocalVarDescs=|Flow rate into the chamber (m^3/s)|Pressure at the inlet (Pa)|Output torque (N*m)|Shaft angular velocity (rad/s)|Power (W)  LocalVarLogging=[0 0 0 0 0]
  Rotational Damper : fl_lib/Mechanical/Rotational Elements/Rotational Damper  Orientation=left  DialogController=NetworkEngine.DynNeDlgSource  SystemSampleTime=-1  D=Damping_Coef N*m/(rad/s)  torque_Log=off  velocity_Log=off  power_Log=off  LocalVarNames=|torque|velocity|power  LocalVarDescs=|Damping torque (N*m)|Damper relative velocity (rad/s)|Power dissipated in the damper (W)  LocalVarLogging=[0 0 0]
  Rotational Hard Stop : fl_lib/Mechanical/Rotational Elements/Rotational Hard Stop  Orientation=left  DialogController=NetworkEngine.DynNeDlgSource  SystemSampleTime=-1  upper_bnd=stroke - init_pos rad  lower_bnd=-init_pos rad  stiff_up=stiffness N*m/rad  stiff_neg=stiffness N*m/rad  D_up=damping N*m/(rad/s)  D_low=damping N*m/(rad/s)  contact_torque_Log=off  rel_angle_Log=off  LocalVarNames=|contact_torque|rel_angle  LocalVarDescs=|Contact torque (N*m)|Slider-case relative angle (rad)  LocalVarLogging=[0 0]
  A : PMIOPort  Tag=PMCPort  Port=1  Side=Left
  B : PMIOPort  Tag=PMCPort  Orientation=left  Port=2  Side=Left
  C : PMIOPort  Tag=PMCPort  Port=3  Side=Right
  S : PMIOPort  Tag=PMCPort  Orientation=left  Port=4  Side=Right
  connections:
  S/RConn1 -- Rotational Hard Stop/LConn1 -- Rotational Hydro-Mechanical Converter/RConn1 -- Rotational Hydro-Mechanical Converter1/RConn1 -- Rotational Damper/LConn1
  Rotational Hydro-Mechanical Converter/LConn1 -- C/RConn1 -- Rotational Hydro-Mechanical Converter1/LConn1 -- Rotational Hard Stop/RConn1 -- Rotational Damper/RConn1
  A/RConn1 -- Rotational Hydro-Mechanical Converter/LConn2
  B/RConn1 -- Rotational Hydro-Mechanical Converter1/LConn2

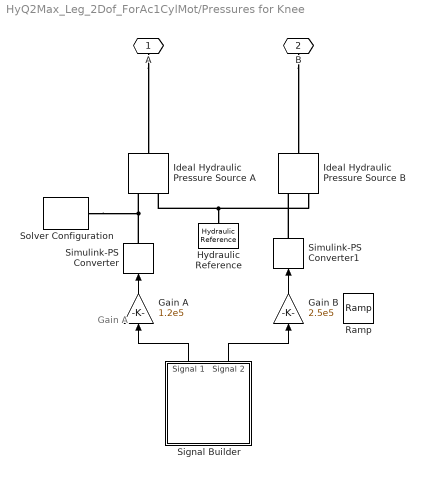
== system HyQ2Max_Leg_2Dof_ForAc1CylMot/Pressures for Knee ==
  note: Gain A
  Gain A : Gain  Orientation=up  Gain=1.2e5  ParameterDataType=sfix(16)  ParameterScaling=2^0  OutDataType=sfix(16)  OutScaling=2^0
  Gain B : Gain  Orientation=up  Gain=2.5e5  ParameterDataType=sfix(16)  ParameterScaling=2^0  OutDataType=sfix(16)  OutScaling=2^0
  Hydraulic Reference : fl_lib/Hydraulic/Hydraulic Elements/Hydraulic Reference  Orientation=down  DialogController=NetworkEngine.DynNeDlgSource  SystemSampleTime=-1  LocalVarLogging=[]
  Ideal Hydraulic Pressure Source A : fl_lib/Hydraulic/Hydraulic Sensors and Sources/Ideal Hydraulic Pressure Source  Orientation=down  DialogController=NetworkEngine.DynNeDlgSource  SystemSampleTime=-1  flow_rate_Log=off  pr_differential_Log=off  power_Log=off  LocalVarNames=|flow_rate|pr_differential|power  LocalVarDescs=|Flow rate through the source (m^3/s)|Pressure differential across the source (Pa)|Source power (W)  LocalVarLogging=[0 0 0]
  Ideal Hydraulic Pressure Source B : fl_lib/Hydraulic/Hydraulic Sensors and Sources/Ideal Hydraulic Pressure Source  Orientation=down  DialogController=NetworkEngine.DynNeDlgSource  SystemSampleTime=-1  flow_rate_Log=off  pr_differential_Log=off  power_Log=off  LocalVarNames=|flow_rate|pr_differential|power  LocalVarDescs=|Flow rate through the source (m^3/s)|Pressure differential across the source (Pa)|Source power (W)  LocalVarLogging=[0 0 0]
  Ramp : simulink/Sources/Ramp  Orientation=left  SystemSampleTime=-1  slope=1  start=1  X0=0
  Signal Builder : Subsystem  Tag=STV Subsys  Orientation=up  LoadFcn=sigbuilder_block('load');  StartFcn=sigbuilder_block('start');  StopFcn=sigbuilder_block('stop');  ClipboardFcn=sigbuilder_block('clipboard');  mask(Sigbuilder block){}
      mask help: Sigbuilder GUI
      mask init:
      | if ~strcmp(get_param(bdroot(gcbh),'SimulationStatus'),'stopped') tuvar = sigbuilder_block('maskInit'); end
      settings: CopyFcn=sigbuilder_block('copy');  DeleteFcn=sigbuilder_block('delete');  ModelCloseFcn=sigbuilder_block('modelClose');  PreSaveFcn=sigbuilder_block('preSave');  NameChangeFcn=sigbuilder_block('namechange');  OpenFcn=sigbuilder_block('open',[388.5 359.25 550.5 371.25 ]);  CloseFcn=sigbuilder_block('close');
      mask Display: plot(0,0,100,100,[10,10,40,40,10],[80,20,20,80,80],[40,10],[50,50], [40,27,10],[65,72,56],[40,25,25,10],[28,28,43,43]);
  Simulink-PS Converter : nesl_utility/Simulink-PS Converter  Orientation=up  DialogController=NetworkEngine.DynNeUtilDlgSource  SystemSampleTime=-1  PhysicalDomain=network_engine_domain  LeftPortType=input  RightPortType=output  SubClassName=ps_input  Unit=N/m^2
  Simulink-PS Converter1 : nesl_utility/Simulink-PS Converter  Orientation=up  DialogController=NetworkEngine.DynNeUtilDlgSource  SystemSampleTime=-1  PhysicalDomain=network_engine_domain  LeftPortType=input  RightPortType=output  SubClassName=ps_input  Unit=N/m^2
  Solver Configuration : nesl_utility/Solver Configuration  DialogController=NetworkEngine.DynNeUtilDlgSource  SystemSampleTime=-1  PhysicalDomain=network_engine_domain  LeftPortType=input  RightPortType=generic  SubClassName=solver  ResidualTolerance=1e-9  MaxNonlinIter=12  MaxModeIter=2  DoFixedCost=off  DoDC=on  LinearAlgebra=Full  Accelerate=off
  A : PMIOPort  Orientation=down  Port=1  Side=Right
  B : PMIOPort  Orientation=down  Port=2  Side=Left
  wires:
  Signal Builder/1(Signal 1) -> Gain A/1
  Gain A/1 -> Simulink-PS Converter/1
  Gain B/1 -> Simulink-PS Converter1/1
  Signal Builder/2(Signal 2) -> Gain B/1
  connections:
  Simulink-PS Converter/RConn1 -- Ideal Hydraulic Pressure Source A/RConn1 -- Solver Configuration/RConn1
  Simulink-PS Converter1/RConn1 -- Ideal Hydraulic Pressure Source B/RConn1
  A/RConn1 -- Ideal Hydraulic Pressure Source A/LConn1
  B/RConn1 -- Ideal Hydraulic Pressure Source B/LConn1
  Ideal Hydraulic Pressure Source B/RConn2 -- Ideal Hydraulic Pressure Source A/RConn2 -- Hydraulic Reference/LConn1

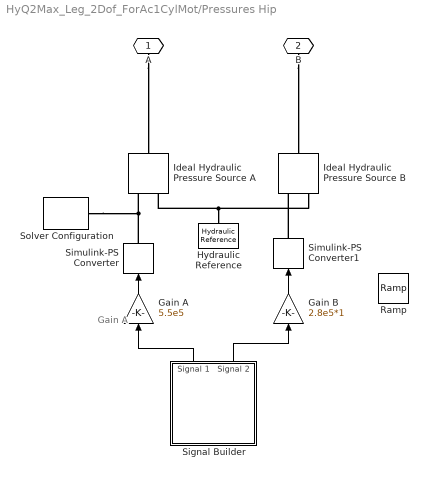
== system HyQ2Max_Leg_2Dof_ForAc1CylMot/Pressures Hip ==
  note: Gain A
  Gain A : Gain  Orientation=up  Gain=5.5e5  ParameterDataType=sfix(16)  ParameterScaling=2^0  OutDataType=sfix(16)  OutScaling=2^0
  Gain B : Gain  Orientation=up  Gain=2.8e5*1  ParameterDataType=sfix(16)  ParameterScaling=2^0  OutDataType=sfix(16)  OutScaling=2^0
  Hydraulic Reference : fl_lib/Hydraulic/Hydraulic Elements/Hydraulic Reference  Orientation=down  DialogController=NetworkEngine.DynNeDlgSource  SystemSampleTime=-1  LocalVarLogging=[]
  Ideal Hydraulic Pressure Source A : fl_lib/Hydraulic/Hydraulic Sensors and Sources/Ideal Hydraulic Pressure Source  Orientation=down  DialogController=NetworkEngine.DynNeDlgSource  SystemSampleTime=-1  flow_rate_Log=off  pr_differential_Log=off  power_Log=off  LocalVarNames=|flow_rate|pr_differential|power  LocalVarDescs=|Flow rate through the source (m^3/s)|Pressure differential across the source (Pa)|Source power (W)  LocalVarLogging=[0 0 0]
  Ideal Hydraulic Pressure Source B : fl_lib/Hydraulic/Hydraulic Sensors and Sources/Ideal Hydraulic Pressure Source  Orientation=down  DialogController=NetworkEngine.DynNeDlgSource  SystemSampleTime=-1  flow_rate_Log=off  pr_differential_Log=off  power_Log=off  LocalVarNames=|flow_rate|pr_differential|power  LocalVarDescs=|Flow rate through the source (m^3/s)|Pressure differential across the source (Pa)|Source power (W)  LocalVarLogging=[0 0 0]
  Ramp : simulink/Sources/Ramp  Orientation=left  SystemSampleTime=-1  slope=1  start=1  X0=0
  Signal Builder : Subsystem  Tag=STV Subsys  Orientation=up  LoadFcn=sigbuilder_block('load');  StartFcn=sigbuilder_block('start');  StopFcn=sigbuilder_block('stop');  ClipboardFcn=sigbuilder_block('clipboard');  mask(Sigbuilder block){}
      mask help: Sigbuilder GUI
      mask init:
      | if ~strcmp(get_param(bdroot(gcbh),'SimulationStatus'),'stopped') tuvar = sigbuilder_block('maskInit'); end
      settings: CopyFcn=sigbuilder_block('copy');  DeleteFcn=sigbuilder_block('delete');  ModelCloseFcn=sigbuilder_block('modelClose');  PreSaveFcn=sigbuilder_block('preSave');  NameChangeFcn=sigbuilder_block('namechange');  OpenFcn=sigbuilder_block('open',[388.5 359.25 550.5 371.25 ]);  CloseFcn=sigbuilder_block('close');
      mask Display: plot(0,0,100,100,[10,10,40,40,10],[80,20,20,80,80],[40,10],[50,50], [40,27,10],[65,72,56],[40,25,25,10],[28,28,43,43]);
  Simulink-PS Converter : nesl_utility/Simulink-PS Converter  Orientation=up  DialogController=NetworkEngine.DynNeUtilDlgSource  SystemSampleTime=-1  PhysicalDomain=network_engine_domain  LeftPortType=input  RightPortType=output  SubClassName=ps_input  Unit=N/m^2
  Simulink-PS Converter1 : nesl_utility/Simulink-PS Converter  Orientation=up  DialogController=NetworkEngine.DynNeUtilDlgSource  SystemSampleTime=-1  PhysicalDomain=network_engine_domain  LeftPortType=input  RightPortType=output  SubClassName=ps_input  Unit=N/m^2
  Solver Configuration : nesl_utility/Solver Configuration  DialogController=NetworkEngine.DynNeUtilDlgSource  SystemSampleTime=-1  PhysicalDomain=network_engine_domain  LeftPortType=input  RightPortType=generic  SubClassName=solver  ResidualTolerance=1e-9  MaxNonlinIter=12  MaxModeIter=2  DoFixedCost=off  DoDC=on  LinearAlgebra=Full  Accelerate=off
  A : PMIOPort  Orientation=down  Port=1  Side=Right
  B : PMIOPort  Orientation=down  Port=2  Side=Left
  wires:
  Signal Builder/1(Signal 1) -> Gain A/1
  Gain A/1 -> Simulink-PS Converter/1
  Gain B/1 -> Simulink-PS Converter1/1
  Signal Builder/2(Signal 2) -> Gain B/1
  connections:
  Simulink-PS Converter/RConn1 -- Ideal Hydraulic Pressure Source A/RConn1 -- Solver Configuration/RConn1
  Simulink-PS Converter1/RConn1 -- Ideal Hydraulic Pressure Source B/RConn1
  A/RConn1 -- Ideal Hydraulic Pressure Source A/LConn1
  B/RConn1 -- Ideal Hydraulic Pressure Source B/LConn1
  Ideal Hydraulic Pressure Source B/RConn2 -- Ideal Hydraulic Pressure Source A/RConn2 -- Hydraulic Reference/LConn1

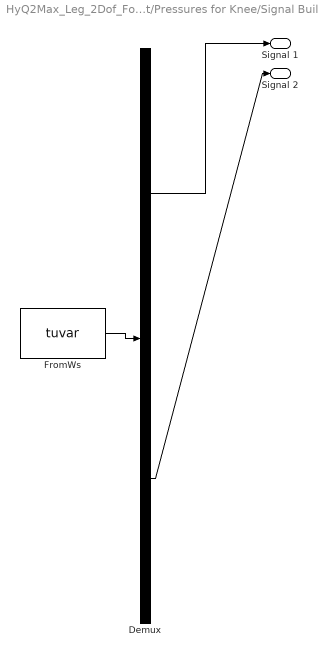
== system HyQ2Max_Leg_2Dof_ForAc1CylMot/Pressures for Knee/Signal Builder ==
  Demux : Demux  Tag=STV Demux  Outputs=2
  FromWs : FromWorkspace  Tag=STV FromWs  VariableName=tuvar  SampleTime=0  SigBuilderData=DataTag1  VnvData=DataTag2
      SigBuilderData=|
      | channels(1).label = 'Signal 1'
      | channels(1).allXData = {[0 1.02 4 5 6 7 8.02 10]}
      | channels(1).allYData = {[0 0 0.01 0.79 1 0.79 0.01 0]}
      | channels(2).label = 'Signal 2'
      | channels(2).allXData = {[0 1.02 1.02 2 3 4 5.02 10]}
      | channels(2).allYData = {[0 0 0.01 0.79 1 0.79 0.01 0]}
      | common.afterFinalStr = 'Extrapolate'
      | common.sampleTime = 0
      | dataSet.timeRange = [0 10]
      | dataSet.name = 'Group 1'
  Signal 1 : Outport  Tag=STV Outport  OutDataType=sfix(16)  OutScaling=2^0
  Signal 2 : Outport  Tag=STV Outport  Port=2  OutDataType=sfix(16)  OutScaling=2^0
  wires:
  Demux/1 -> Signal 1/1
  FromWs/1 -> Demux/1
  Demux/2 -> Signal 2/1

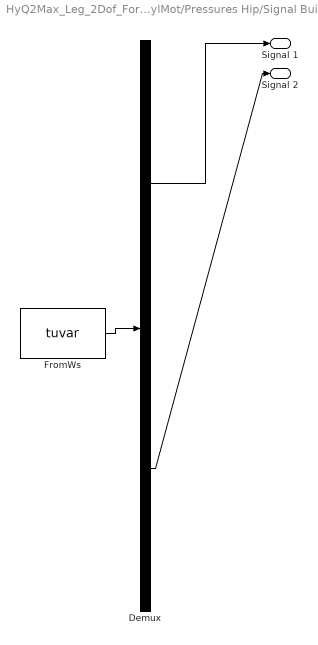
== system HyQ2Max_Leg_2Dof_ForAc1CylMot/Pressures Hip/Signal Builder ==
  Demux : Demux  Tag=STV Demux  Outputs=2
  FromWs : FromWorkspace  Tag=STV FromWs  VariableName=tuvar  SampleTime=0  SigBuilderData=DataTag3  VnvData=DataTag4
      SigBuilderData=|
      | channels(1).label = 'Signal 1'
      | channels(1).allXData = {[0 1.02 1.02 2 3 4 5.02 10]}
      | channels(1).allYData = {[0 0 0.01 0.79 1 0.79 0.01 0]}
      | channels(2).label = 'Signal 2'
      | channels(2).allXData = {[0 4 5 5.98 6.98 7.98 10]}
      | channels(2).allYData = {[0 0 0.79 0.997010505051 0.78 0 0]}
      | common.afterFinalStr = 'Extrapolate'
      | common.sampleTime = 0
      | dataSet.timeRange = [0 10]
      | dataSet.name = 'Group 1'
  Signal 1 : Outport  Tag=STV Outport  OutDataType=sfix(16)  OutScaling=2^0
  Signal 2 : Outport  Tag=STV Outport  Port=2  OutDataType=sfix(16)  OutScaling=2^0
  wires:
  Demux/1 -> Signal 1/1
  FromWs/1 -> Demux/1
  Demux/2 -> Signal 2/1
